simulink model "robotsimulation"  (R2021b)
settings: Solver=ode3  StartTime=0.0  StopTime=2  FixedStep=0.001  MaxStep=0.01  RelTol=1e-2
values from neighbouring files (symbols this model uses):
  fext = zeros(6,8)    [simIRB120.m]    (also in simIRB120_nofriction.m)
  fv = [.1,.1,.1,.05,.05,.05]    [simIRB120.m]    (also in simIRB120_nofriction.m)
  kd = [  20;   20;   10;  0.5;   0.5; 0.05]    [simIRB120.m]    (also in simIRB120_nofriction.m)
  ki = [  65;  100;  300;   .5;   0.5;   .1]    [simIRB120.m]    (also in simIRB120_nofriction.m)
  kp = [  20;  150;  450; 3.55;     5;  .75]    [simIRB120.m]    (also in simIRB120_nofriction.m)
  qdes = (rand(6,1)-.5)*2*pi    [simIRB120.m]    (also in simIRB120_nofriction.m)
  qdotinit = zeros(6,1)    [simIRB120.m]    (also in simIRB120_nofriction.m)
  qinit = zeros(6,1)    [simIRB120.m]    (also in simIRB120_nofriction.m)
libraries: simulink x1, robotmaniplib x1, slpidlib x1
settings Model: Creator=wen  LastModifiedBy=Yuxin
settings SolverCC: ZeroCrossAlgorithm=Adaptive  AlgebraicLoopSolver=TrustRegion
settings DebuggingCC: IgnoredZcDiagnostic=none  SFMachineParentedDataDiag=warning

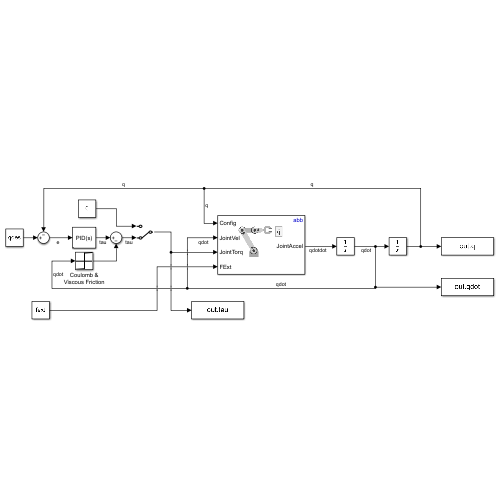
[thumbnail: Simulink's stored preview of the top-level diagram]
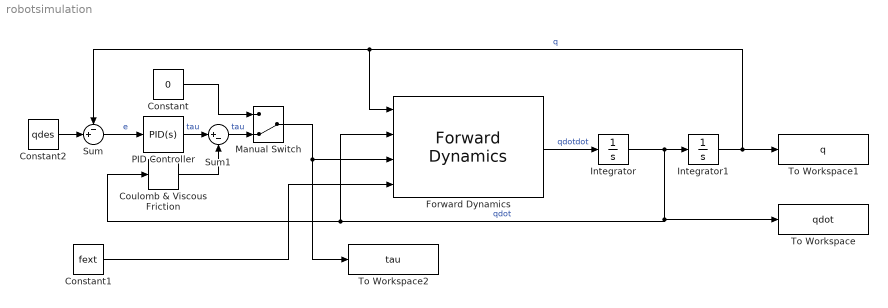
== system robotsimulation ==
  Constant : Constant  Value=0
  Constant1 : Constant  Value=fext
  Constant2 : Constant  Value=qdes
  Coulomb & Viscous Friction : simulink/Discontinuities/Coulomb & Viscous Friction  offset=fc  gain=fv
  Forward Dynamics : robotmaniplib/Forward Dynamics  RigidBodyTree=abb  SimulateUsing=Interpreted execution
  Integrator : Integrator  InitialCondition=qdotinit
  Integrator1 : Integrator  InitialCondition=qinit
  Manual Switch : ManualSwitch  CurrentSetting=0
  PID Controller : slpidlib/PID Controller  Controller=PID  Form=Parallel  TimeDomain=Continuous-time  UseExternalTs=off  SampleTime=-1  IntegratorMethod=Forward Euler  FilterMethod=Forward Euler  ControllerParametersSource=internal  P=kp  I=ki  D=kd  UseFilter=on  N=100  TunerSelectOption=Transfer Function Based (PID Tuner App)  InitialConditionSource=internal  InitialConditionForIntegrator=0  InitialConditionForFilter=0  DifferentiatorICPrevScaledInput=0  ExternalReset=none  TrackingMode=off  Kt=1  LimitOutput=off  SatLimitsSource=internal  UpperSaturationLimit=inf  LowerSaturationLimit=-inf  LinearizeAsGain=on  AntiWindupMode=none  Kb=1  POutMin=[]  POutMax=[]  IOutMin=[]  IOutMax=[]  DOutMin=[]  DOutMax=[]  NOutMin=[]  NOutMax=[]  SumOutMin=[]  SumOutMax=[]  SaturationOutMin=[]  SaturationOutMax=[]  PParamMin=[]  PParamMax=[]  IParamMin=[]  IParamMax=[]  DParamMin=[]  DParamMax=[]  NParamMin=[]  NParamMax=[]  KbParamMin=[]  KbParamMax=[]  KtParamMin=[]  KtParamMax=[]  KbOutMin=[]  KbOutMax=[]  KtOutMin=[]  KtOutMax=[]  IntegratorOutMin=[]  IntegratorOutMax=[]  FilterOutMin=[]  FilterOutMax=[]  SumI1OutMin=[]  SumI1OutMax=[]  SumI2OutMin=[]  SumI2OutMax=[]  SumI3OutMin=[]  SumI3OutMax=[]  SumI4OutMin=[]  SumI4OutMax=[]  SumDOutMin=[]  SumDOutMax=[]  DifferentiatorOutMin=[]  DifferentiatorOutMax=[]  FilterDiffOutCoefMin=[]  FilterDiffOutCoefMax=[]  ReciprocalOutMin=[]  ReciprocalOutMax=[]  SumDenOutMin=[]  SumDenOutMax=[]  SumNumOutMin=[]  SumNumOutMax=[]  DivideOutMin=[]  DivideOutMax=[]  UdiffTsProdOutMin=[]  UdiffTsProdOutMax=[]  NTsProdOutMin=[]  NTsProdOutMax=[]  UintegralTsProdOutMin=[]  UintegralTsProdOutMax=[]  UngainTsProdOutMin=[]  UngainTsProdOutMax=[]  IntegratorContinuousStateAttributes=''  IntegratorStateMustResolveToSignalObject=off  IntegratorRTWStateStorageClass=Auto  FilterContinuousStateAttributes=''  FilterStateMustResolveToSignalObject=off  FilterRTWStateStorageClass=Auto  ParallelPVariant=InternalParameters  IdealPVariant=Disabled  IVariant=InternalParameters  DVariant=InternalParameters  IntegratorVariant=Continuous  SatVariant=Disabled  AWVariant=Passthrough  PCopyVariant=Disabled  TRVariant=Disabled  FdbkBlocksVariant=Forward  IdealPFdbkVariant=Disabled  SatFdbkVariant=Disabled  DerivativeFilterVariant=ContFilter  NVariant=InternalParameters  NCopyVariant=Disabled  FilterICVariant=InternalICsFilter  IntegratorICVariant=InternalICs  ExternalResetVariant=Disabled  TRSumVariant=Passthrough  SumFdbkVariant=Disabled  SumVariant=Sum_PID  TsampFilterVariant=InternalTs  TsampNgainVariant=Passthrough  TsampIntegralVariant=Passthrough  ExternalSaturationOutDataTypeStr=Inherit: Same as second input
  Sum : Sum  Inputs=-+|
  Sum1 : Sum  Inputs=|+-
  To Workspace : ToWorkspace  VariableName=qdot  SampleTime=-1
  To Workspace1 : ToWorkspace  VariableName=q  SampleTime=-1
  To Workspace2 : ToWorkspace  VariableName=tau  SampleTime=-1
      settings: Save2DSignal=2-D array (concatenate along first dimension)
  wires:
  Forward Dynamics/1 -> Integrator/1  "qdotdot"
  Integrator/1 -> Forward Dynamics/2, Coulomb & Viscous Friction/1, To Workspace/1, Integrator1/1  "qdot"
  Integrator1/1 -> Forward Dynamics/1, Sum/1, To Workspace1/1  "q"
  Constant1/1 -> Forward Dynamics/4
  Sum/1 -> PID Controller/1  "e"
  Constant2/1 -> Sum/2
  PID Controller/1 -> Sum1/1  "tau"
  Coulomb & Viscous Friction/1 -> Sum1/2
  Manual Switch/1 -> To Workspace2/1, Forward Dynamics/3
  Sum1/1 -> Manual Switch/2  "tau"
  Constant/1 -> Manual Switch/1
